simulink model "LQR"  (R2023a)
settings: Solver=VariableStepAuto  StartTime=0.0  StopTime=30  RelTol=1e-3
settings Model: Creator=c  LastModifiedBy=c

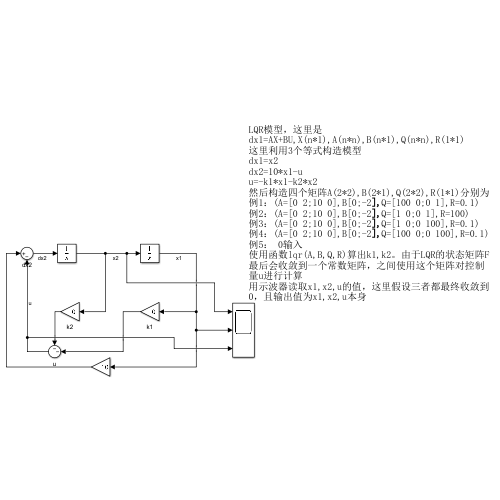
[thumbnail: Simulink's stored preview of the top-level diagram]
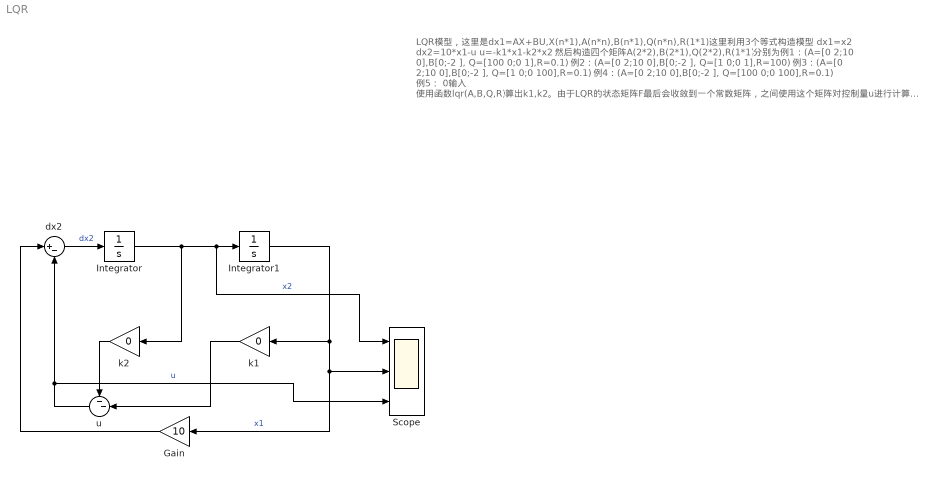
== system LQR ==
  note: LQR模型，这里是dx1=AX+BU,X(n*1),A(n*n),B(n*1),Q(n*n),R(1*1)
      | 这里利用3个等式构造模型
      | dx1=x2
      | dx2=10*x1-u
      | u=-k1*x1-k2*x2
      | 然后构造四个矩阵A(2*2),B(2*1),Q(2*2),R(1*1)分别为例1：(A=[0 2;10 0],B[0;-2 ], Q=[100 0;0 1],R=0.1)
      | 例2：(A=[0 2;10 0],B[0;-2 ], Q=[1 0;0 1],R=100)
      | 例3：(A=[0 2;10 0],B[0;-2 ], Q=[1 0;0 100],R=0.1)
      | 例4：(A=[0 2;10 0],B[0;-2 ], Q=[100 0;0 100],R=0.1)
      | 例5： 0输入
      | 使用函数lqr(A,B,Q,R)算出k1,k2。由于LQR的状态矩阵F最后会收敛到一个常数矩阵，之间使用这个矩阵对控制量u进行计算
      | 用示波器读取x1,x2,u的值，这里假设三者都最终收敛到0，且输出值为x1,x2,u本身
  Gain : Gain  Gain=10
  Integrator : Integrator
  Integrator1 : Integrator  InitialCondition=5
  Scope : Scope  NumInputPorts=3
  dx2 : Sum  Inputs=|+-
  k1 : Gain  Gain=0
  k2 : Gain  Gain=0
  u : Sum  Inputs=--|
  wires:
  Integrator/1 -> k2/1, Scope/1, Integrator1/1  "x2"
  dx2/1 -> Integrator/1  "dx2"
  Integrator1/1 -> Gain/1, Scope/2, k1/1  "x1"
  k2/1 -> u/1
  k1/1 -> u/2
  u/1 -> dx2/2, Scope/3  "u"
  Gain/1 -> dx2/1
